simulink model "PARITY_checker_odd_even_manual_bit_updating"  (R2021b)
settings: Solver=VariableStepAuto  StartTime=0.0  StopTime=10.0  RelTol=1e-3
settings Model: Creator=Joshua  LastModifiedBy=Joshua

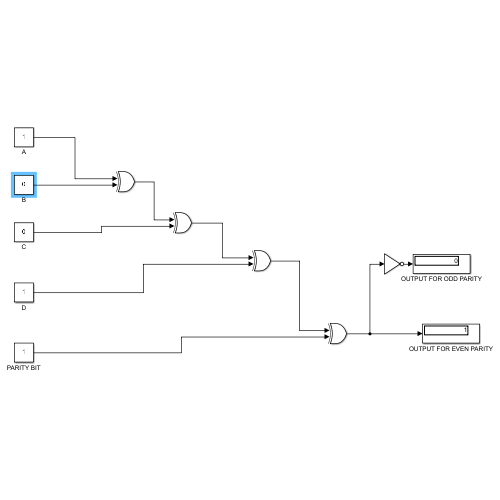
[thumbnail: Simulink's stored preview of the top-level diagram]
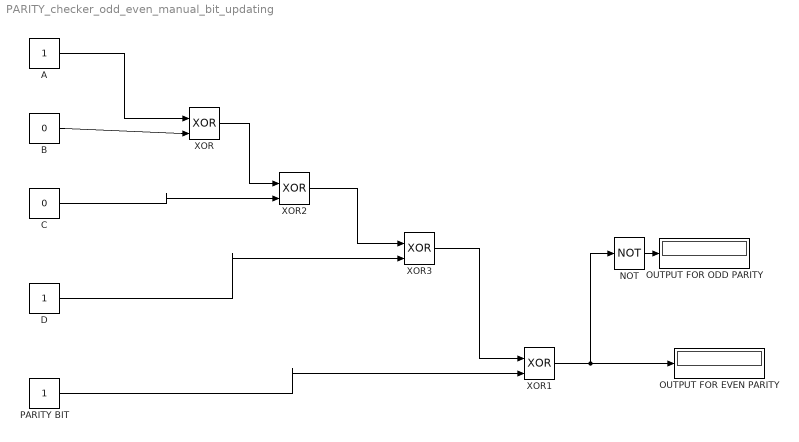
== system PARITY_checker_odd_even_manual_bit_updating ==
  A : Constant
  B : Constant  Value=0
  C : Constant  Value=0
  D : Constant
  NOT : Logic  Operator=NOT  IconShape=distinctive  AllPortsSameDT=off  OutDataTypeStr=boolean
  OUTPUT FOR EVEN PARITY : Display
  OUTPUT FOR ODD PARITY : Display
  PARITY BIT : Constant
  XOR{,1..3} (4 alike) : Logic  Operator=XOR  IconShape=distinctive  AllPortsSameDT=off  OutDataTypeStr=boolean
  wires:
  XOR1/1 -> OUTPUT FOR EVEN PARITY/1, NOT/1
  XOR3/1 -> XOR1/1
  PARITY BIT/1 -> XOR1/2
  D/1 -> XOR3/2
  C/1 -> XOR2/2
  XOR/1 -> XOR2/1
  A/1 -> XOR/1
  B/1 -> XOR/2
  XOR2/1 -> XOR3/1
  NOT/1 -> OUTPUT FOR ODD PARITY/1
